simulink model "myo_model_architectures"  (R2020b)
settings: Solver=VariableStepAuto  StartTime=0.0  StopTime=10  RelTol=1e-3
undefined symbols (not defined in the file or in its folder): beta_adm, beta_force, beta_force_int, beta_imp, beta_pos, D_adm, J_adm, K_imp, Kd_pos, Kp_pos, posLim, posPole
libraries: cstblocks x36
settings Model: Creator=simon  LastModifiedBy=nicol
settings SolverCC: ZeroCrossAlgorithm=Adaptive
settings DebuggingCC: IgnoredZcDiagnostic=none

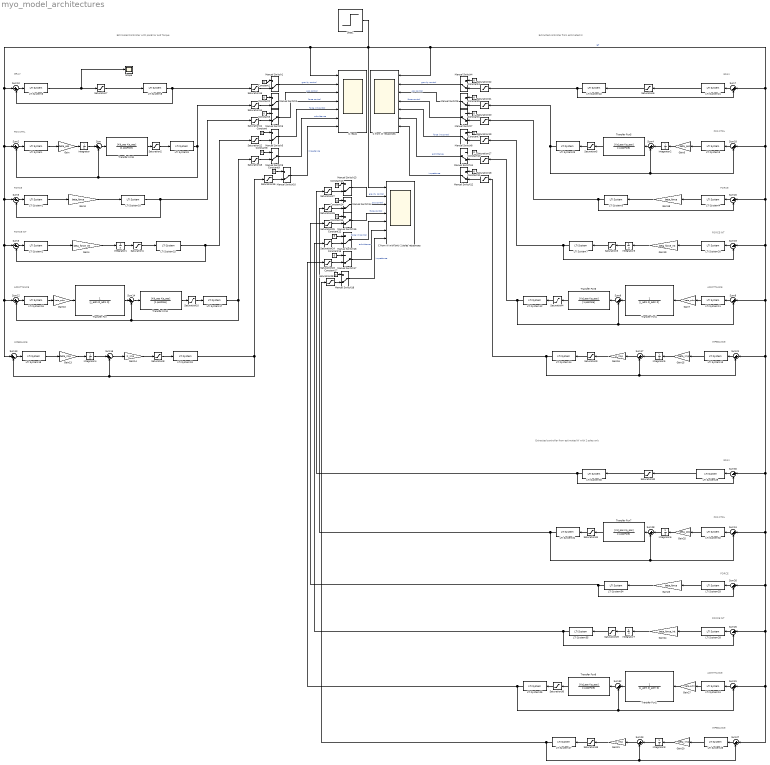
== system myo_model_architectures ==
  note: IMPEDANCE
  note: Estimated Controller with posError and Torque
  note: Extracted controller from estimated W
  note: ADMITTANCE
  note: GRAV
  note: POS CTRL
  note: FORCE
  note: FORCE INT
  note: FORCE
  note: FORCE INT
  note: POS CTRL
  note: IMPEDANCE
  note: ADMITTANCE
  note: GRAV
  note: IMPEDANCE
  note: FORCE INT
  note: POS CTRL
  note: Extracted controller from estimated W with 2 poles only
  note: GRAV
  note: ADMITTANCE
  note: FORCE
  " C resps" : Scope  NumInputPorts=7
  C from W responses : Scope  NumInputPorts=7
  C from W with only 2 poles responses : Scope  NumInputPorts=7
  Constant{,1..17} (18 alike) : Constant  Value=0
  Gain : Gain  Gain=beta_pos
  Gain10 : Gain  Gain=beta_adm
  Gain13 : Gain  Gain=beta_imp
  Gain14 : Gain  Gain=K_imp
  Gain15 : Gain  Gain=beta_imp
  Gain16 : Gain  Gain=K_imp
  Gain18 : Gain  Gain=beta_force
  Gain19 : Gain  Gain=beta_force_int
  Gain20 : Gain  Gain=beta_imp
  Gain21 : Gain  Gain=K_imp
  Gain23 : Gain  Gain=beta_force
  Gain24 : Gain  Gain=beta_force_int
  Gain25 : Gain  Gain=beta_pos
  Gain27 : Gain  Gain=beta_adm
  Gain3 : Gain  Gain=beta_force
  Gain4 : Gain  Gain=beta_force_int
  Gain5 : Gain  Gain=beta_pos
  Gain7 : Gain  Gain=beta_adm
  Integrator{,1..8} (9 alike) : Integrator
  LTI System{,1..2,6,16,18} (6 alike) : cstblocks/LTI System  sys=C_best  IC=[]
  LTI System{5,7..10,12,14..15,17,19,22..23,25,27,30..31,34..35} (18 alike) : cstblocks/LTI System  sys=G_assumed  IC=[]
  LTI System{3..4,11,13,20..21} (6 alike) : cstblocks/LTI System  sys=C_from_Wbest  IC=[]
  LTI System{24,26,28..29,32..33} (6 alike) : cstblocks/LTI System  sys=C_from_W2best  IC=[]
  Manual Switch{1..18} (18 alike) : ManualSwitch  CurrentSetting=0
  Saturation{1..10,29..33} (15 alike) : Saturate  UpperLimit=6  LowerLimit=-6
  Saturation{11..28} (18 alike) : Saturate  UpperLimit=posLim  LowerLimit=-posLim
  Scope : Scope
  Step1 : Step  Time=0  SampleTime=0
  Sum{,2..5,7..10,12..14,16..21,23..28,30..32} (27 alike) : Sum  Inputs=|+-
  Transfer Fcn : TransferFcn  Denominator=[J_adm D_adm 0]
  Transfer Fcn1 : TransferFcn  Denominator=[J_adm D_adm 0]
  Transfer Fcn2 : TransferFcn  Denominator=[J_adm D_adm 0]
  Transfer Fcn{3,5..9} (6 alike) : TransferFcn  Numerator=[Kd_pos Kp_pos]  Denominator=[1 posPole]
  wires:
  Gain/1 -> Integrator/1
  Transfer Fcn9/1 -> Saturation2/1
  Integrator/1 -> Sum/1
  LTI System/1 -> Gain/1
  Sum2/1 -> LTI System/1
  Sum5/1 -> LTI System1/1
  LTI System2/1 -> Gain4/1
  Gain4/1 -> Integrator1/1
  Sum3/1 -> LTI System2/1
  Integrator1/1 -> Saturation1/1
  LTI System1/1 -> Gain3/1
  LTI System6/1 -> Scope/1, Saturation7/1
  Sum10/1 -> LTI System6/1
  Manual Switch1/1 -> " C resps"/2  "gravity control"
  Manual Switch2/1 -> " C resps"/3  "pos control"
  Manual Switch3/1 -> " C resps"/4  "force control"
  Manual Switch5/1 -> " C resps"/5  "force int control"
  Manual Switch4/1 -> C from W responses/2  "gravity control"
  Manual Switch7/1 -> C from W responses/4  "force control"
  Manual Switch6/1 -> C from W responses/3  "pos control"
  Manual Switch8/1 -> C from W responses/5  "force int control"
  Constant/1 -> Manual Switch5/1
  Constant1/1 -> Manual Switch1/1
  Constant2/1 -> Manual Switch2/1
  Constant3/1 -> Manual Switch3/1
  Constant4/1 -> Manual Switch4/1
  Constant5/1 -> Manual Switch6/1
  Constant6/1 -> Manual Switch7/1
  Constant7/1 -> Manual Switch8/1
  LTI System9/1 -> Saturation14/1, Sum/2, Sum2/2
  Saturation2/1 -> LTI System9/1
  LTI System8/1 -> Saturation15/1, Sum10/2
  Saturation7/1 -> LTI System8/1
  LTI System10/1 -> Saturation11/1, Sum5/2
  Gain3/1 -> LTI System10/1
  LTI System15/1 -> Saturation12/1, Sum3/2
  Saturation1/1 -> LTI System15/1
  Sum12/1 -> LTI System16/1
  Saturation8/1 -> LTI System19/1
  Sum13/1 -> LTI System18/1
  LTI System17/1 -> Saturation13/1, Sum12/2, Sum14/2
  Constant8/1 -> Manual Switch9/1
  Constant9/1 -> Manual Switch10/1
  Manual Switch9/1 -> " C resps"/6  "admittance"
  Manual Switch10/1 -> " C resps"/7  "impedance"
  Transfer Fcn3/1 -> Saturation10/1
  LTI System16/1 -> Gain10/1
  Transfer Fcn/1 -> Sum14/1
  Gain10/1 -> Transfer Fcn/1
  Saturation10/1 -> LTI System17/1
  Gain14/1 -> Saturation8/1
  LTI System19/1 -> Saturation16/1, Sum13/2, Sum16/2
  Sum16/1 -> Gain14/1
  Integrator4/1 -> Sum16/1
  Gain13/1 -> Integrator4/1
  LTI System18/1 -> Gain13/1
  Constant11/1 -> Manual Switch12/1
  Manual Switch11/1 -> C from W responses/6  "admittance"
  Manual Switch12/1 -> C from W responses/7  "impedance"
  LTI System13/1 -> Gain15/1
  Gain15/1 -> Integrator5/1
  Integrator5/1 -> Sum17/1
  Gain7/1 -> Transfer Fcn1/1
  Sum8/1 -> LTI System11/1
  Saturation9/1 -> LTI System14/1
  LTI System4/1 -> Gain18/1
  Transfer Fcn1/1 -> Sum9/1
  LTI System5/1 -> Saturation20/1, Sum20/2
  Gain16/1 -> Saturation9/1
  Sum21/1 -> LTI System13/1
  LTI System12/1 -> Saturation17/1, Sum9/2, Sum8/2
  LTI System23/1 -> Saturation21/1, Sum4/2, Sum18/2
  Saturation6/1 -> LTI System22/1
  LTI System20/1 -> Gain19/1
  LTI System22/1 -> Saturation22/1, Sum7/2
  LTI System11/1 -> Gain7/1
  LTI System14/1 -> Saturation18/1, Sum21/2, Sum17/2
  Sum7/1 -> LTI System21/1
  LTI System7/1 -> Saturation19/1, Sum19/2
  Saturation3/1 -> LTI System7/1
  Gain18/1 -> LTI System5/1
  Saturation5/1 -> LTI System23/1
  Sum20/1 -> LTI System4/1
  Integrator3/1 -> Saturation3/1
  Transfer Fcn5/1 -> Saturation5/1
  Sum18/1 -> LTI System3/1
  Sum17/1 -> Gain16/1
  LTI System3/1 -> Gain5/1
  Saturation4/1 -> LTI System12/1
  LTI System21/1 -> Saturation6/1
  Integrator2/1 -> Sum4/1
  Sum19/1 -> LTI System20/1
  Gain5/1 -> Integrator2/1
  Gain19/1 -> Integrator3/1
  Saturation11/1 -> Manual Switch3/2
  Saturation12/1 -> Manual Switch5/2
  Saturation13/1 -> Manual Switch9/2
  Saturation14/1 -> Manual Switch2/2
  Saturation15/1 -> Manual Switch1/2
  Saturation16/1 -> Manual Switch10/2
  Saturation17/1 -> Manual Switch11/2
  Saturation18/1 -> Manual Switch12/2
  Saturation19/1 -> Manual Switch8/2
  Saturation20/1 -> Manual Switch7/2
  Saturation21/1 -> Manual Switch6/2
  Saturation22/1 -> Manual Switch4/2
  LTI System34/1 -> Saturation25/1, Sum26/2
  Gain27/1 -> Transfer Fcn2/1
  Sum28/1 -> Transfer Fcn7/1
  Gain23/1 -> LTI System34/1
  Gain20/1 -> Integrator8/1
  LTI System27/1 -> Saturation28/1, Sum27/2, Sum23/2
  Gain21/1 -> Saturation33/1
  Saturation29/1 -> LTI System35/1
  Sum25/1 -> LTI System28/1
  LTI System35/1 -> Saturation24/1, Sum25/2
  LTI System33/1 -> Gain23/1
  LTI System32/1 -> Gain25/1
  Gain25/1 -> Integrator6/1
  Integrator6/1 -> Sum28/1
  Sum30/1 -> LTI System29/1
  Transfer Fcn2/1 -> Sum32/1
  Saturation31/1 -> LTI System31/1
  Sum23/1 -> Gain21/1
  Sum31/1 -> LTI System24/1
  Sum24/1 -> LTI System32/1
  LTI System26/1 -> Gain20/1
  Saturation30/1 -> LTI System25/1
  Sum26/1 -> LTI System33/1
  LTI System24/1 -> Gain27/1
  Sum27/1 -> LTI System26/1
  LTI System28/1 -> Gain24/1
  Saturation32/1 -> LTI System30/1
  LTI System29/1 -> Saturation32/1
  Saturation33/1 -> LTI System27/1
  LTI System30/1 -> Saturation27/1, Sum30/2
  Gain24/1 -> Integrator7/1
  Integrator7/1 -> Saturation29/1
  LTI System25/1 -> Saturation23/1, Sum32/2, Sum31/2
  Integrator8/1 -> Sum23/1
  Step1/1 -> C from W with only 2 poles responses/1, Sum7/1, Sum20/1, Sum30/1, Sum26/1, Sum27/1, Sum31/1, Sum25/1, Sum24/1, Sum21/1, Sum8/1, Sum19/1, Sum18/1, C from W responses/1, Sum13/1, Sum12/1, Sum3/1, Sum5/1, Sum2/1, Sum10/1, " C resps"/1  "ref"
  LTI System31/1 -> Saturation26/1, Sum28/2, Sum24/2
  Saturation27/1 -> Manual Switch13/2
  Saturation26/1 -> Manual Switch14/2
  Saturation24/1 -> Manual Switch16/2
  Constant15/1 -> Manual Switch15/1
  Saturation23/1 -> Manual Switch17/2
  Constant13/1 -> Manual Switch13/1
  Constant12/1 -> Manual Switch16/1
  Saturation25/1 -> Manual Switch15/2
  Constant16/1 -> Manual Switch17/1
  Constant14/1 -> Manual Switch14/1
  Manual Switch13/1 -> C from W with only 2 poles responses/2  "gravity control"
  Manual Switch14/1 -> C from W with only 2 poles responses/3  "pos control"
  Manual Switch15/1 -> C from W with only 2 poles responses/4  "force control"
  Manual Switch16/1 -> C from W with only 2 poles responses/5  "force int control"
  Manual Switch17/1 -> C from W with only 2 poles responses/6  "admittance"
  Constant17/1 -> Manual Switch18/1
  Saturation28/1 -> Manual Switch18/2
  Manual Switch18/1 -> C from W with only 2 poles responses/7  "impedance"
  Sum/1 -> Transfer Fcn9/1
  Sum14/1 -> Transfer Fcn3/1
  Sum4/1 -> Transfer Fcn5/1
  Transfer Fcn6/1 -> Saturation4/1
  Sum9/1 -> Transfer Fcn6/1
  Transfer Fcn7/1 -> Saturation31/1
  Transfer Fcn8/1 -> Saturation30/1
  Sum32/1 -> Transfer Fcn8/1
